simulink model "Askhsh_7"  (R2018b)
settings: Solver=VariableStepAuto  StartTime=0.0  StopTime=15  RelTol=1e-3
undefined symbols (not defined in the file): sigbuilder_block
settings Model: Creator=mluser  LastModifiedBy=Argy
settings DataIOCC: ReturnWorkspaceOutputs=on  Refine=10
settings DebuggingCC: UnconnectedInputMsg=none  UnconnectedOutputMsg=none  UnconnectedLineMsg=none
settings ModelReferenceCC: EnableRefExpFcnMdlSchedulingChecks=off
settings RTWCC: Description=Generic Real-Time Target

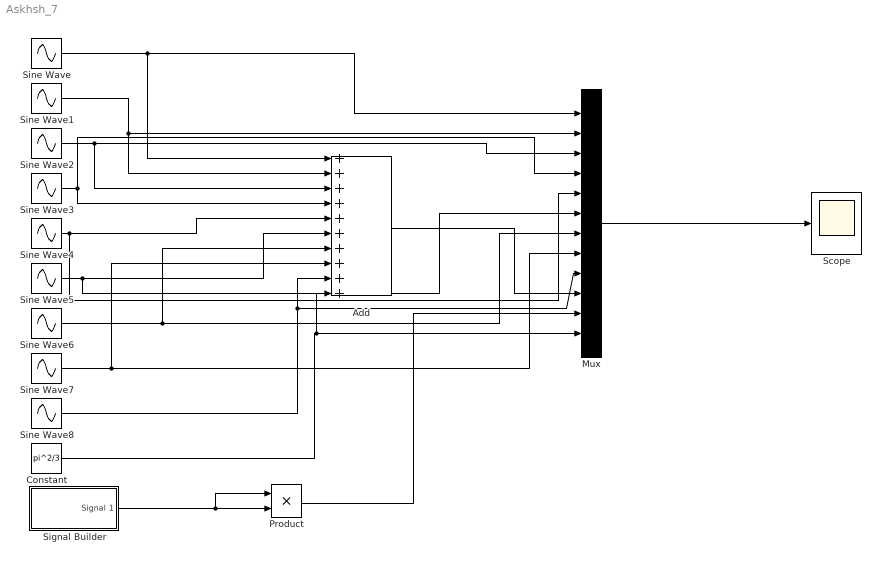
== system Askhsh_7 ==
  Add : Sum  Inputs=++++++++++
  Constant : Constant  Value=pi^2/3
  Mux : Mux  Inputs=12
  Product : Product
  Scope : Scope
  Signal Builder : Subsystem  Tag=STV Subsys  LoadFcn=sigbuilder_block('load');  StartFcn=sigbuilder_block('start');  StopFcn=sigbuilder_block('stop');  ClipboardFcn=sigbuilder_block('clipboard');  mask(Sigbuilder block){tuvar=[0:10]}
      mask help: Simulink:masks:SigbuilderBlock_MD
      mask init:
      | if ~strcmp(get_param(bdroot(gcbh),'SimulationStatus'),'stopped') tuvar = sigbuilder_block('maskInit'); end
      settings: CopyFcn=sigbuilder_block('copy');  DeleteFcn=sigbuilder_block('delete');  ModelCloseFcn=sigbuilder_block('modelClose');  PreSaveFcn=sigbuilder_block('preSave');  PauseFcn=sigbuilder_block('pause');  ContinueFcn=sigbuilder_block('continue');  NameChangeFcn=sigbuilder_block('namechange');  OpenFcn=sigbuilder_block('open',[0 30 1152 561.6 ]);  CloseFcn=sigbuilder_block('close');
      mask Display: plot(0, 0, 100, 100,[2, 2, 32, 32, 2], [68, 8, 8, 68, 68],[32, 2], [38, 38], [32, 19, 2],[53, 60, 44], [32, 17, 17, 2],[16, 16, 31, 31]);txt = getActiveGroup(gcbh);text(2, 100, txt,'verticalAlignment', 'top');
  Sine Wave : Sin  Amplitude=-4  Phase=pi/2  SampleTime=0
  Sine Wave1 : Sin  Frequency=2  Phase=pi/2  SampleTime=0
  Sine Wave2 : Sin  Amplitude=-4/9  Frequency=3  Phase=pi/2  SampleTime=0
  Sine Wave3 : Sin  Amplitude=1/4  Frequency=4  Phase=pi/2  SampleTime=0
  Sine Wave4 : Sin  Amplitude=-4/25  Frequency=5  Phase=pi/2  SampleTime=0
  Sine Wave5 : Sin  Amplitude=4/36  Frequency=6  Phase=pi/2  SampleTime=0
  Sine Wave6 : Sin  Amplitude=-4/49  Frequency=7  Phase=pi/2  SampleTime=0
  Sine Wave7 : Sin  Amplitude=4/64  Frequency=8  Phase=pi/2  SampleTime=0
  Sine Wave8 : Sin  Amplitude=-4/81  Frequency=9  Phase=pi/2  SampleTime=0
  wires:
  Mux/1 -> Scope/1
  Signal Builder/1(Signal 1) -> Product/1, Product/2
  Sine Wave1/1 -> Mux/2, Add/2
  Sine Wave2/1 -> Mux/3, Add/3
  Sine Wave4/1 -> Mux/5, Add/5
  Sine Wave5/1 -> Mux/6, Add/6
  Sine Wave6/1 -> Mux/7, Add/7
  Sine Wave7/1 -> Mux/8, Add/8
  Sine Wave8/1 -> Mux/9, Add/9
  Sine Wave3/1 -> Add/4, Mux/4
  Product/1 -> Mux/11
  Add/1 -> Mux/10
  Sine Wave/1 -> Add/1, Mux/1
  Constant/1 -> Add/10, Mux/12

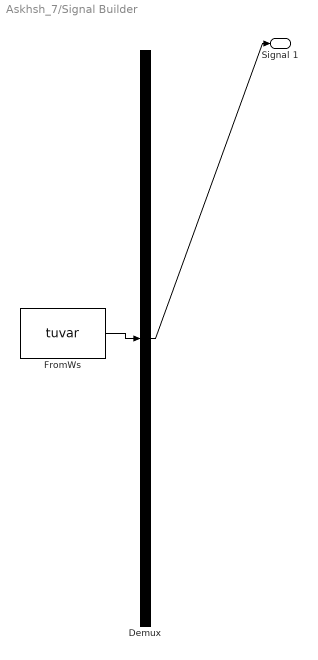
== system Askhsh_7/Signal Builder ==
  Demux : Demux  Tag=STV Demux  Outputs=1
  FromWs : FromWorkspace  Tag=STV FromWs  VariableName=tuvar  SampleTime=0
      SigBuilderData=|
      | common.afterFinalStr = 'Extrapolate'
      | common.sampleTime = 0
      | dataSet.timeRange = [0 12.5663706144]
      | dataSet.name = 'Group 1'
      | sbobj.Groups.Name = 'Group 1'
      | sbobj.Groups.Signals.Name = 'Signal 1'
      | sbobj.Groups.Signals.XData = [0 3.14159265359 6.28319 9.42477796077 12.5663706144]
      | sbobj.Groups.Signals.YData = [0 3.14159265359 0 3.14159265359 0]
      | sbobj.Groups.TimeRange = [0 12.5663706144]
  Signal 1 : Outport  Tag=STV Outport
  wires:
  FromWs/1 -> Demux/1
  Demux/1 -> Signal 1/1
